simulink model "obliczeniaOffline"  (R2013a)
settings: Solver=FixedStepDiscrete  StartTime=0  StopTime=15  FixedStep=0.0025  RelTol=1e-3
InitFcn:
  | InitFcn
values from neighbouring files (symbols this model uses):
  accBias = zeros(3,1)    [InitFcn.m]
  accGain = accGain.*(9.81/9.761)    [InitFcn.m]
  gyroBias = zeros(3,1)    [InitFcn.m]
  gyroGain = ones(3,1)    [InitFcn.m]
  index = 1    [InitFcn.m]
  magBias = [(743-502);(743-507);(579-516)]/2    [InitFcn.m]
  magGainM = W_inverted    [InitFcn.m]
  usrednien = 5    [InitFcn.m]
undefined symbols (not defined in the file or in its folder): dfilt, DiscIntNeverNeededParam, eul_0, fdesignblkfcn, gcbh
libraries: dspstat3 x12, aerolibconvert2 x9, aerolibobsolete x7, aerolibtransform2 x4, dspmtrx3 x3, aerolibutil x3, dspsigops x1, dspsrcs4 x1, dsparch4 x1
settings Model: Creator=Antonio  LastModifiedBy=Antonio
settings SolverCC: AutoInsertRateTranBlk=on  InsertRTBMode=Always
settings OptimizationCC: LocalBlockOutputs=off  SimCompilerOptimization=On
settings SFSimCC: SFSimEnableDebug=off
settings RTWCC: RTWCompilerOptimization=On

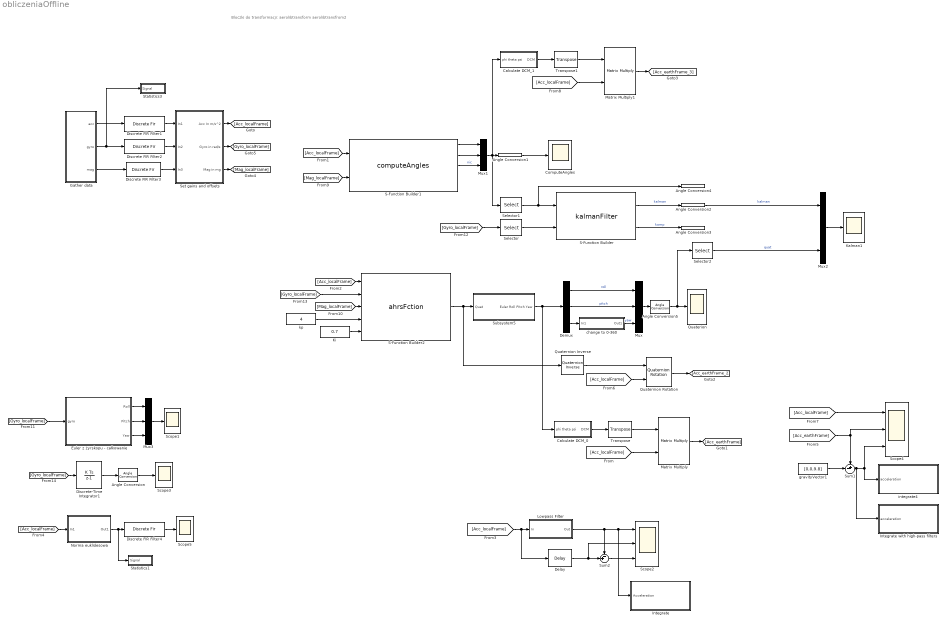
== system obliczeniaOffline ==
  note: Bloczki do transformacji:
      | aerolibtransform
      | aerolibtransfrom2
  " Set gains and offsets" : Subsystem
  Angle Conversion{,1..5} (6 alike) : aerolibconvert2/Angle Conversion  IU=rad  OU=deg
  Calculate DCM_0 : Subsystem
  Calculate DCM_1 : Subsystem
  ComputeAngles : Scope
      settings: TickLabels=on  ShowLegends=on  TimeRange=30  YMin=-125  YMax=375  SaveName=ScopeData3
  Delay : dspsigops/Delay  dly_unit=Samples  delay=0  ic_detail=off  dif_ic_for_ch=off  dif_ic_for_dly=off  ic=0  reset_popup=None
  Demux : Demux  Outputs=3
  Discrete FIR Filter1 : DiscreteFir  Coefficients=ones(1,usrednien)/usrednien
  Discrete FIR Filter2 : DiscreteFir  Coefficients=ones(1,usrednien)/usrednien
  Discrete FIR Filter3 : DiscreteFir  Coefficients=ones(1,usrednien)/usrednien
  Discrete FIR Filter4 : DiscreteFir  Coefficients=ones(1,15)/15
  Discrete-Time Integrator1 : DiscreteIntegrator  SampleTime=-1  ICPrevOutput=DiscIntNeverNeededParam  ICPrevScaledInput=DiscIntNeverNeededParam
  Euler z żyrskopu - całkowanie : Subsystem
  Gather data : Subsystem
  Integrate : Subsystem
  Integrate with high-pass filters : Subsystem
  Kalman1 : Scope
      settings: ShowLegends=on  TimeRange=15  YMin=-10  YMax=180  SaveName=ScopeData5
  Ki : Constant  Value=0.7  OutDataTypeStr=single
  Lowpass Filter : Subsystem  DialogController=fdesignblkfcn  InitFcn=fdesignblkfcn(gcbh, {'InitFcn'});  mask(Lowpass Filter){}
      mask help: Design a lowpass filter
      settings: CopyFcn=fdesignblkfcn(gcbh, {'CopyFcn'});
      mask Help: helpview(mapfilelocation('dsp'), 'dsplowpassfilter');
      mask Display: disp('Lowpass')
  Matrix Multiply : Product  Multiplication=Matrix(*)
  Matrix Multiply1 : Product  Multiplication=Matrix(*)
  Mux{,1..3} (4 alike) : Mux  Inputs=3
  Norma euklidesowa : Subsystem
  Quaterion : Scope
      settings: ShowLegends=on  TimeRange=15  YMin=-25  YMax=375  SaveName=ScopeData4
  Quaternion Inverse : aerolibutil/Quaternion Inverse
  Quaternion Rotation : aerolibutil/Quaternion Rotation
  S-Function Builder : S-Function  InitFcn=try, set_param(gcb,'FunctionName','kalmanFilter'), end  FunctionName=kalmanFilter  Parameters=single(0.0025)  SFunctionModules=kalmanFilter_wrapper Kalman  EnableBusSupport=off  mask(S-Function Builder){}
      mask help: Simulink:masks:SFunctionBuilder_MD
      mask init:
      | val = [[.9  0.75 0.75 1 1 .9 .9 1]',[1 1 0.75 0.75 .9 .9 1 .9]'];try , sys = get_param(gcb,'SfunBuilderFcnName');if isempty(sys), sys = get_param(gcb,'FunctionName'); end,catch, sys = get_param(gcb,'FunctionName'); end
      settings: CopyFcn=set_param(gcbh,'LinkStatus','none')  PreSaveFcn=try, set_param(gcb,'FunctionName','kalmanFilter'), end  OpenFcn=sfunctionwizard(gcbh)
      mask Display: plot(val(:,1),val(:,2)),disp(sys), port_label('input',1,'newAngleIn'), port_label('input',2,'newRateIn'), port_label('output',1,'angleOut'), port_label('output',2,'compAngleOut')
  S-Function Builder1 : S-Function  InitFcn=try, set_param(gcb,'FunctionName','computeAngles'), end  FunctionName=computeAngles  SFunctionModules=computeAngles_wrapper angles  EnableBusSupport=off  mask(S-Function Builder){}
      mask help: Simulink:masks:SFunctionBuilder_MD
      mask init: same as obliczeniaOffline/S-Function Builder
      settings: CopyFcn=set_param(gcbh,'LinkStatus','none')  PreSaveFcn=try, set_param(gcb,'FunctionName','computeAngles'), end  OpenFcn=sfunctionwizard(gcbh)
      mask Display: plot(val(:,1),val(:,2)),disp(sys), port_label('input',1,'accelerometerIn'), port_label('input',2,'magnetometerIn'), port_label('output',1,'XRollAngleOut'), port_label('output',2,'YPitchAngleOut'), port_label('output',3,'ZYawAngleOut'), port_label('output',4,'ZYawAngleFlatOut'), port_label('output',5,'TiltAngleOut')
  S-Function Builder2 : S-Function  InitFcn=try, set_param(gcb,'FunctionName','ahrsFction'), end  FunctionName=ahrsFction  SFunctionModules=ahrsFction_wrapper artykul MahonyAHRS  EnableBusSupport=off  mask(S-Function Builder){}
      mask help: Simulink:masks:SFunctionBuilder_MD
      mask init: same as obliczeniaOffline/S-Function Builder
      settings: CopyFcn=set_param(gcbh,'LinkStatus','none')  PreSaveFcn=try, set_param(gcb,'FunctionName','ahrsFction'), end  OpenFcn=sfunctionwizard(gcbh)
      mask Display: plot(val(:,1),val(:,2)),disp(sys), port_label('input',1,'accIn'), port_label('input',2,'gyroIn'), port_label('input',3,'magIn'), port_label('input',4,'Kp'), port_label('input',5,'Ki'), port_label('output',1,'quat')
  Scope1 : Scope
      settings: ShowLegends=on  TimeRange=60  YMin=-3  YMax=3
  Scope2 : Scope  NumInputPorts=3
      settings: ShowLegends=on  TimeRange=15  YMin=-2~-5~-4  YMax=10~15~10  SaveName=ScopeData2
  Scope3 : Scope
      settings: ShowLegends=on  TimeRange=60  YMin=-350  YMax=50  SaveName=ScopeData6
  Scope4 : Scope  NumInputPorts=3
      settings: ShowLegends=on  TimeRange=15  YMin=-2.03431~-2~-2  YMax=11.8546~11~1.75  SaveName=ScopeData8
  Scope5 : Scope
      settings: ShowLegends=on  TimeRange=60  YMin=2  YMax=11  SaveName=ScopeData11
  Selector : Selector  InputPortWidth=3  IndexOptions=Index vector (dialog)  Indices=[index]  OutputSizes=1
  Selector1 : Selector  InputPortWidth=3  IndexOptions=Index vector (dialog)  Indices=[index]  OutputSizes=1
  Selector2 : Selector  InputPortWidth=3  IndexOptions=Index vector (dialog)  Indices=[index]  OutputSizes=1
  Statistics1 : Subsystem
  Statistics3 : Subsystem
  Subsystem5 : Subsystem
  Sum1 : Sum  Inputs=+-|
  Sum2 : Sum  Inputs=-+|
  Transpose : dspmtrx3/Transpose  Hermitian=off  overflowFlag=off
  Transpose1 : dspmtrx3/Transpose  Hermitian=off  overflowFlag=off
  change to 0-360 : Subsystem
  gravityVector1 : Constant  Value=[0,0,9.8]
  integrate4 : Subsystem
  kp : Constant  Value=4  OutDataTypeStr=single
  wires:
  Selector/1 -> S-Function Builder/2
  Gather data/1(acc) -> Discrete FIR Filter1/1
  Gather data/2(gyro) -> Discrete FIR Filter2/1, Statistics3/1(Signal)
  Gather data/3(mag) -> Discrete FIR Filter3/1
  Discrete FIR Filter2/1 -> " Set gains and offsets"/2(In2)
  Discrete FIR Filter3/1 -> " Set gains and offsets"/3(In3)
  Mux2/1 -> Kalman1/1
  Mux/1 -> Angle Conversion5/1
  Demux/3 -> change to 0-360/1(In1)
  change to 0-360/1(Out1) -> Mux/3  "yaw"
  Demux/2 -> Mux/2  "pitch"
  Demux/1 -> Mux/1  "roll"
  S-Function Builder1/2 -> Mux1/2
  S-Function Builder1/3 -> Mux1/3  "nic"
  S-Function Builder1/1 -> Mux1/1
  Selector1/1 -> Angle Conversion4/1, S-Function Builder/1
  Angle Conversion1/1 -> ComputeAngles/1
  Euler z żyrskopu - całkowanie/1(Roll) -> Mux3/1
  Euler z żyrskopu - całkowanie/2(Pitch) -> Mux3/2
  Euler z żyrskopu - całkowanie/3(Yaw) -> Mux3/3
  Mux3/1 -> Scope1/1
  Selector2/1 -> Mux2/3  "quat"
  S-Function Builder/2 -> Angle Conversion3/1  "komp"
  S-Function Builder/1 -> Angle Conversion2/1  "kalman"
  Discrete-Time Integrator1/1 -> Angle Conversion/1
  Angle Conversion/1 -> Scope3/1
  Mux1/1 -> Calculate DCM_1/1(phi theta psi), Selector1/1, Angle Conversion1/1
  kp/1 -> S-Function Builder2/4
  Ki/1 -> S-Function Builder2/5
  Calculate DCM_0/1(DCM) -> Transpose/1
  Subsystem5/1(Euler Roll Pitch Yaw) -> Demux/1, Calculate DCM_0/1(phi theta psi)
  Angle Conversion2/1 -> Mux2/1  "kalman"
  Transpose/1 -> Matrix Multiply/1
  [Acc_localFrame] -> Matrix Multiply/2
  gravityVector1/1 -> Sum1/2
  Matrix Multiply/1 -> [Acc_earthFrame]
  S-Function Builder2/1 -> Quaternion Inverse/1, Subsystem5/1(Quat)
  [Acc_localFrame] -> S-Function Builder1/1
  [Acc_localFrame] -> S-Function Builder2/1
  Quaternion Inverse/1 -> Quaternion Rotation/1
  Sum2/1 -> Scope2/3
  [Acc_localFrame] -> Lowpass Filter/1(In), Delay/1
  Delay/1 -> Scope2/2, Sum2/2
  Norma euklidesowa/1(Out1) -> Statistics1/1(Signal), Discrete FIR Filter4/1
  [Acc_localFrame] -> Norma euklidesowa/1(In1)
  Angle Conversion5/1 -> Selector2/1, Quaterion/1
  [Acc_earthFrame] -> Sum1/1, Scope4/2
  [Acc_localFrame] -> Quaternion Rotation/2
  Quaternion Rotation/1 -> [Acc_earthFrame_2]
  [Acc_localFrame] -> Scope4/1
  Discrete FIR Filter1/1 -> " Set gains and offsets"/1(In1)
  Lowpass Filter/1(Out) -> Integrate/1(Acceleration), Scope2/1, Sum2/1
  Discrete FIR Filter4/1 -> Scope5/1
  " Set gains and offsets"/1(Acc In m/s^2) -> [Acc_localFrame]
  Sum1/1 -> Integrate with high-pass filters/1(acceleration), integrate4/1(acceleration), Scope4/3
  Calculate DCM_1/1(DCM) -> Transpose1/1
  Transpose1/1 -> Matrix Multiply1/1
  [Acc_localFrame] -> Matrix Multiply1/2
  Matrix Multiply1/1 -> [Acc_earthFrame_3]
  " Set gains and offsets"/3(Mag in mg) -> [Mag_localFrame]
  [Mag_localFrame] -> S-Function Builder1/2
  [Mag_localFrame] -> S-Function Builder2/3
  " Set gains and offsets"/2(Gyro in rad/s) -> [Gyro_localFrame]
  [Gyro_localFrame] -> Euler z żyrskopu - całkowanie/1(gyro)
  [Gyro_localFrame] -> Selector/1
  [Gyro_localFrame] -> S-Function Builder2/2
  [Gyro_localFrame] -> Discrete-Time Integrator1/1

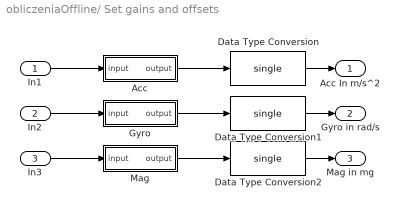
== system obliczeniaOffline/ Set gains and offsets ==
  In1 : Inport
  In2 : Inport  Port=2
  In3 : Inport  Port=3
  Acc : Subsystem
  Data Type Conversion : DataTypeConversion  OutDataTypeStr=single
  Data Type Conversion1 : DataTypeConversion  OutDataTypeStr=single
  Data Type Conversion2 : DataTypeConversion  OutDataTypeStr=single
  Gyro : Subsystem
  Mag : Subsystem
  Acc In m/s^2 : Outport
  Gyro in rad/s : Outport  Port=2
  Mag in mg : Outport  Port=3
  wires:
  Gyro/1(output) -> Data Type Conversion1/1
  In3/1 -> Mag/1(input)
  In2/1 -> Gyro/1(input)
  Acc/1(output) -> Data Type Conversion/1
  In1/1 -> Acc/1(input)
  Mag/1(output) -> Data Type Conversion2/1
  Data Type Conversion/1 -> Acc In m/s^2/1
  Data Type Conversion1/1 -> Gyro in rad/s/1
  Data Type Conversion2/1 -> Mag in mg/1

== system obliczeniaOffline/Calculate DCM_0 ==
  phi theta psi : Inport
  Rotation Angles to Direction Cosine Matrix : aerolibtransform2/Rotation Angles to Direction Cosine Matrix  rotationOrder=ZYX
  Selector : Selector  InputPortWidth=3  IndexOptions=Index vector (dialog)  Indices=[3 2 1]  OutputSizes=1
  DCM : Outport
  wires:
  Selector/1 -> Rotation Angles to Direction Cosine Matrix/1
  phi theta psi/1 -> Selector/1
  Rotation Angles to Direction Cosine Matrix/1 -> DCM/1

== system obliczeniaOffline/Calculate DCM_1 ==
  phi theta psi : Inport
  Rotation Angles to Direction Cosine Matrix : aerolibtransform2/Rotation Angles to Direction Cosine Matrix  rotationOrder=ZYX
  Selector : Selector  InputPortWidth=3  IndexOptions=Index vector (dialog)  Indices=[3 2 1]  OutputSizes=1
  DCM : Outport
  wires:
  Selector/1 -> Rotation Angles to Direction Cosine Matrix/1
  phi theta psi/1 -> Selector/1
  Rotation Angles to Direction Cosine Matrix/1 -> DCM/1

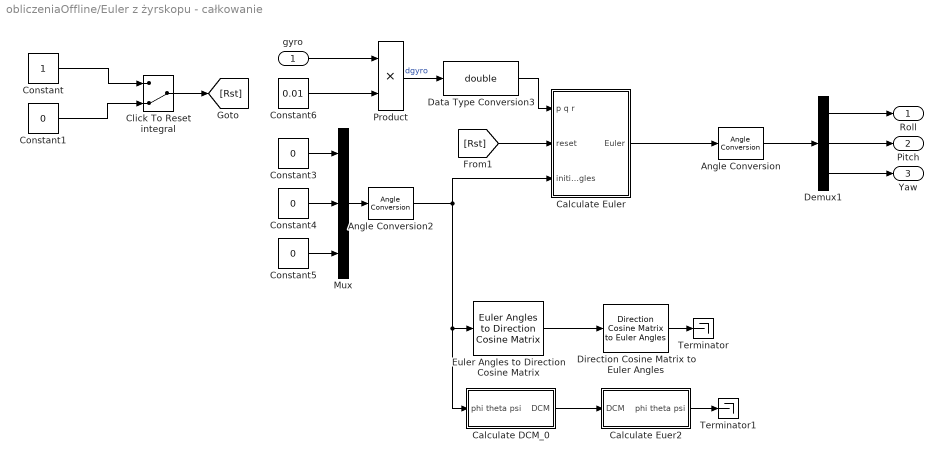
== system obliczeniaOffline/Euler z żyrskopu - całkowanie ==
  gyro : Inport
  Angle Conversion : aerolibconvert2/Angle Conversion  IU=rad  OU=deg
  Angle Conversion2 : aerolibconvert2/Angle Conversion  IU=deg  OU=rad
  Calculate DCM_0 : Subsystem
  Calculate Euer2 : Subsystem
  Calculate Euler : Subsystem
  Click To Reset integral : ManualSwitch  CurrentSetting=0
  Constant : Constant
  Constant{1,3..5} (4 alike) : Constant  Value=0
  Constant6 : Constant  Value=0.01  OutDataTypeStr=single
  Data Type Conversion3 : DataTypeConversion  OutDataTypeStr=double
  Demux1 : Demux  Outputs=3
  Direction Cosine Matrix to Euler Angles : aerolibobsolete/Direction Cosine Matrix to Euler Angles
  Euler Angles to Direction Cosine Matrix : aerolibobsolete/Euler Angles to  Direction Cosine Matrix
  Mux : Mux  Inputs=3
  Product : Product
  Terminator : Terminator
  Terminator1 : Terminator
  Roll : Outport
  Pitch : Outport  Port=2
  Yaw : Outport  Port=3
  wires:
  Constant/1 -> Click To Reset integral/1
  Constant1/1 -> Click To Reset integral/2
  Click To Reset integral/1 -> [Rst]
  Calculate Euler/1(Euler) -> Angle Conversion/1
  Demux1/2 -> Pitch/1
  Demux1/1 -> Roll/1
  Demux1/3 -> Yaw/1
  Angle Conversion/1 -> Demux1/1
  Constant3/1 -> Mux/1
  Constant4/1 -> Mux/2
  Constant5/1 -> Mux/3
  Mux/1 -> Angle Conversion2/1
  [Rst] -> Calculate Euler/2(reset)
  Angle Conversion2/1 -> Calculate Euler/3(initialAngles), Calculate DCM_0/1(phi theta psi), Euler Angles to Direction Cosine Matrix/1
  Constant6/1 -> Product/2
  Product/1 -> Data Type Conversion3/1  "dgyro"
  Euler Angles to Direction Cosine Matrix/1 -> Direction Cosine Matrix to Euler Angles/1
  Calculate DCM_0/1(DCM) -> Calculate Euer2/1(DCM)
  Data Type Conversion3/1 -> Calculate Euler/1(p q r)
  gyro/1 -> Product/1
  Direction Cosine Matrix to Euler Angles/1 -> Terminator/1
  Calculate Euer2/1(phi theta psi) -> Terminator1/1

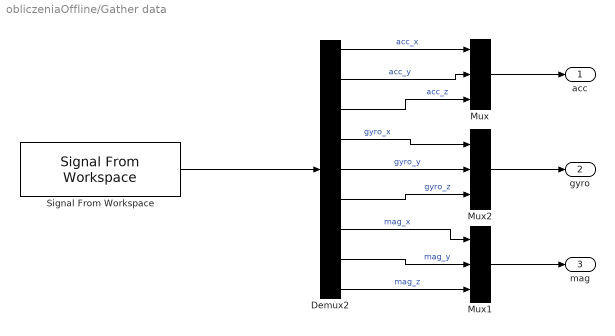
== system obliczeniaOffline/Gather data ==
  Demux2 : Demux  Outputs=9
  Mux : Mux  Inputs=3
  Mux1 : Mux  Inputs=3
  Mux2 : Mux  Inputs=3
  Signal From Workspace : dspsrcs4/Signal From Workspace  X=measurement  Ts=0.0025  nsamps=1  OutputAfterFinalValue=Holding final value  ignoreOrWarnInputAndFrameLengths=off
  acc : Outport
  gyro : Outport  Port=2
  mag : Outport  Port=3
  wires:
  Demux2/1 -> Mux/1  "acc_x"
  Demux2/2 -> Mux/2  "acc_y"
  Demux2/3 -> Mux/3  "acc_z"
  Mux/1 -> acc/1
  Demux2/5 -> Mux2/2  "gyro_y"
  Demux2/4 -> Mux2/1  "gyro_x"
  Demux2/6 -> Mux2/3  "gyro_z"
  Mux2/1 -> gyro/1
  Demux2/7 -> Mux1/1  "mag_x"
  Demux2/8 -> Mux1/2  "mag_y"
  Demux2/9 -> Mux1/3  "mag_z"
  Mux1/1 -> mag/1
  Signal From Workspace/1 -> Demux2/1

== system obliczeniaOffline/Integrate ==
  Acceleration : Inport
  Discrete-Time Integrator2 : DiscreteIntegrator  gainval=1  SampleTime=-1  ICPrevOutput=DiscIntNeverNeededParam  ICPrevScaledInput=DiscIntNeverNeededParam
  Discrete-Time Integrator3 : DiscreteIntegrator  gainval=1  SampleTime=-1  ICPrevOutput=DiscIntNeverNeededParam  ICPrevScaledInput=DiscIntNeverNeededParam
  Product : Product
  Step : Step  Time=5
  m to cm : Gain  Gain=100
  pozycja : Scope  NumInputPorts=3
      settings: ShowLegends=on  TimeRange=15  YMin=-15~-500~-0.4  YMax=15~4750~0.05  SaveName=ScopeData10
  wires:
  Discrete-Time Integrator2/1 -> pozycja/2, Discrete-Time Integrator3/1  "velocity"
  Discrete-Time Integrator3/1 -> pozycja/3  "position"
  Product/1 -> m to cm/1
  Acceleration/1 -> Product/1
  Step/1 -> Product/2
  m to cm/1 -> Discrete-Time Integrator2/1, pozycja/1

== system obliczeniaOffline/Integrate with high-pass filters ==
  acceleration : Inport
  Discrete-Time Integrator2 : DiscreteIntegrator  gainval=1  SampleTime=-1  ICPrevOutput=DiscIntNeverNeededParam  ICPrevScaledInput=DiscIntNeverNeededParam
  Discrete-Time Integrator3 : DiscreteIntegrator  gainval=0.5  SampleTime=-1  ICPrevOutput=DiscIntNeverNeededParam  ICPrevScaledInput=DiscIntNeverNeededParam
  Highpass Filter2 : Subsystem  DialogController=fdesignblkfcn  InitFcn=fdesignblkfcn(gcbh, {'InitFcn'});  mask(Highpass Filter){}
      mask help: Design a highpass filter
      settings: CopyFcn=fdesignblkfcn(gcbh, {'CopyFcn'});
      mask Help: helpview(mapfilelocation('dsp'), 'dsphighpassfilter');
      mask Display: disp('Highpass')
  Product : Product
  Step : Step  Time=5
  m to cm : Gain  Gain=100
  pozycja : Scope  NumInputPorts=3
      settings: ShowLegends=on  TimeRange=15  YMin=-150~-25~-30  YMax=150~25~20  SaveName=ScopeData10
  wires:
  Discrete-Time Integrator2/1 -> pozycja/2, Discrete-Time Integrator3/1  "velocity"
  Discrete-Time Integrator3/1 -> pozycja/3  "position"
  Product/1 -> m to cm/1
  acceleration/1 -> Product/1
  Step/1 -> Product/2
  Highpass Filter2/1(Out) -> pozycja/1, Discrete-Time Integrator2/1
  m to cm/1 -> Highpass Filter2/1(In)

== system obliczeniaOffline/Lowpass Filter ==
  In : Inport
  Generated Filter Block : DiscreteFir  Tag=BlockMethodSubSystem  Coefficients=[0.00050680699585200345 1.8104768139348693e-05 1.6977561331381059e-05 1.4833633469184346e-05 1.1634485977210355e-05 7.3434816185162684e-06 1.925238505602481e-06 -4.6554062756843208e-06 -1.2428942588863933e-05 -2.14243220317547e-05 -3.1665536877958055e-05 -4.3173212468487982e-05 -5.596345481140389e-05 -7.0045256722031624e-05 -8.5422243813193955e-05 -0.0001020913503340876 -0.00012004374546061746 -0.0001392619546353783 -0.00015972622688413584 -0.00018138836919694775 -0.00020423491202698217 -0.00022818978603687275 -0.00025320269989232124 -0.00027921558906226688 -0.00030614886036985707 -0.00033391218088171478 -0.00036241524341515939 -0.00039155711714154967 -0.00042123049572248105 -0.00045131620561162018 -0.00048168727910416389 -0.00051221020993199337 -0.00054274521301832886 -0.00057314784243304084 -0.00060326880695485527 -0.00063295356901068699 -0.00066204167658164611 -0.00069037270007361678 -0.00071777933332873526 -0.00074410555802311438 -0.00076918180057893579 -0.00079284492083031837 -0.00081493914228260192 -0.00083530657953818509 -0.00085378919210934404 -0.00087024715251888445 -0.00088453633553146611 -0.00089652433072802298 -0.00090608418959002091 -0.00091310030908900691 -0.00091746820875369787 -0.00091909427196526061 -0.00091789573503021709 -0.00091380214009601022 -0.00090675563447802381 -0.00089671236011365518 -0.00088364731133413999 -0.00086754948936208873 -0.00084842749881238876 -0.00082629818291407955 -0.00080119748719947067 -0.00077319086865142021 -0.0007423606677744815 -0.00070877954903689048 -0.00067258226676091047 -0.00063388601583306409 -0.00059284204523740128 -0.00054961325206677003 -0.00050437902638090885 -0.00045733140230810318 -0.00040867457706862047 -0.00035862264400760783 -0.00030740039285116294 -0.00025524021333557913 -0.00020238061194014591 -0.00014906827871743485 -9.555603919256272e-05 -4.2109642615560943e-05 1.0990394190089968e-05 6.3432131552027015e-05 0.00011481508771645329 0.000163929526711354 0.00021337941369384917 0.00026014518432284408 0.00030496071711733048 0.00034749727121142219 0.00038749962497370752 0.00042472979420425259 0.00045896558094866979 0.00048999762759601795 0.00051763444976912288 0.00054170106937079287 0.00056204277991718878 0.00057852591164379548 0.00059103671920925928 0.00059948483928015488 0.00060380313045349618 0.00060395022421946181 0.0005999086230995391 0.00059169306814376116 0.00057931861944241988 0.00056288200358844227 0.00054243478381470699 0.00051810065614346363 0.00049002865769549658 0.00045837773939839727 0.0004233288051232909 0.00038509540043196559 0.00034391229856337252 0.00030003785456418733 0.00025374627222805494 0.0002053296340389396 0.00015509716876202419 0.00010337338110347834 5.0497602022540693e-05 -3.1789803530603983e-06 -5.7296714938403917e-05 -0.00011149165215694587 -0.00016539253821891225 -0.00021863218629743133 -0.00027082953146300635 -0.0003216221132869809 -0.00037064610713815347 -0.00041754058093965694 -0.00046196133091381565 -0.00050358116726620307 -0.00054207560146992545 -0.00057714811813586371 -0.00060851810603824888 -0.00063593013978642055 -0.00065915071230361502 -0.00067797096142335322 -0.00069220947241619779 -0.00070171458496094436 -0.00070636537888095789 -0.00070607362183796652 -0.00070078440447933759 -0.00069047251380168991 -0.00067514898155686962 -0.00065485547577851465 -0.0006296782561620325 -0.00059973710746372762 -0.00056517563643030462 -0.00052617404653279305 -0.00048297031526965364 -0.00043579580170031166 -0.00038494458296995683 -0.00033072396635073088 -0.00027347214432053829 -0.00021354989195547714 -0.00015134089229504571 -8.7248797179902441e-05 -2.1695978491134758e-05 4.4880429387894182e-05 0.00011202804206761498 0.00017927981156929496 0.00024615815775456187 0.00031217479280710493 0.00037684128493064596 0.00043967486237110029 0.00050021947128286873 0.0005580848283111197 0.00061307792246632106 0.0006639966539519446 0.00071116167118856575 0.000753898713209556 0.00079188230416504021 0.00082478164102509045 0.0008522956280890945 0.00087415501109185589 ...(+15061 chars)]
  Out : Outport
  wires:
  In/1 -> Generated Filter Block/1
  Generated Filter Block/1 -> Out/1

== system obliczeniaOffline/Norma euklidesowa ==
  In1 : Inport
  Matrix Multiply1 : Product  Multiplication=Matrix(*)
  Sqrt : Sqrt  SaturateOnIntegerOverflow=on
  Transpose1 : dspmtrx3/Transpose  Hermitian=off  overflowFlag=off
  Out1 : Outport
  wires:
  Transpose1/1 -> Matrix Multiply1/1
  In1/1 -> Matrix Multiply1/2, Transpose1/1
  Matrix Multiply1/1 -> Sqrt/1
  Sqrt/1 -> Out1/1

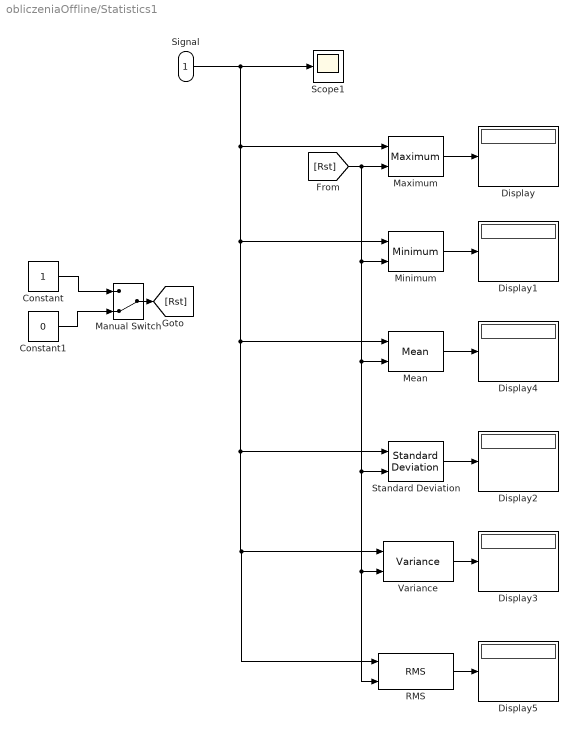
== system obliczeniaOffline/Statistics1 ==
  Signal : Inport
  Constant : Constant
  Constant1 : Constant  Value=0
  Display{,1..5} (6 alike) : Display
  Manual Switch : ManualSwitch  CurrentSetting=0
  Maximum : dspstat3/Maximum  fcn=Running  reset=Either edge  indexBase=One  operateOver=Each column  Dimension=1  colComp=on  operation=maximum  roiEnable=off  roiType=Rectangles  roiPortion=Entire ROI  roiOutput=Individual statistics for each ROI  roiFlag=off  accumDataTypeStr=Inherit: Same as product output  accumLastDataTypeStr=Inherit: Same as product output  roundingMode=Floor  overflowMode=off
  Mean : dspstat3/Mean  run=on  reset_popup=Either edge  directionMode=Each column  dimension=1  treatSBRowAsCol=on  roiEnable=off  roiType=Rectangles  roiPortion=Entire ROI  roiOutput=Individual statistics for each ROI  roiFlag=off  outputDataTypeStr=Inherit: Same as accumulator  outputLastDataTypeStr=Inherit: Same as accumulator  outputMin=[]  outputMax=[]  roundingMode=Floor  overflowMode=off
  Minimum : dspstat3/Minimum  fcn=Running  reset=Either edge  indexBase=One  operateOver=Each column  Dimension=1  colComp=on  operation=minimum  roiEnable=off  roiType=Rectangles  roiPortion=Entire ROI  roiOutput=Individual statistics for each ROI  roiFlag=off  roundingMode=Floor  overflowMode=off
  RMS : dspstat3/RMS  run=on  reset_popup=Either edge  directionMode=Each column  dimension=1  treatSBRowAsCol=on
  Scope1 : Scope
      settings: ShowLegends=on  TimeRange=50  YMin=-40000  YMax=40000
  Standard Deviation : dspstat3/Standard Deviation  run=on  reset_popup=Either edge  directionMode=Each column  dimension=1  treatSBRowAsCol=on  roiEnable=off  roiType=Rectangles  roiPortion=Entire ROI  roiOutput=Individual statistics for each ROI  roiFlag=off
  Variance : dspstat3/Variance  run=on  reset_popup=Either edge  directionMode=Each column  dimension=1  treatSBRowAsCol=on  roiEnable=off  roiType=Rectangles  roiPortion=Entire ROI  roiOutput=Individual statistics for each ROI  roiFlag=off  roundingMode=Floor  overflowMode=off
  wires:
  Variance/1 -> Display3/1
  Constant/1 -> Manual Switch/1
  Standard Deviation/1 -> Display2/1
  Constant1/1 -> Manual Switch/2
  Minimum/1 -> Display1/1
  Manual Switch/1 -> [Rst]
  Maximum/1 -> Display/1
  Signal/1 -> Scope1/1, Mean/1, RMS/1, Variance/1, Standard Deviation/1, Minimum/1, Maximum/1
  Mean/1 -> Display4/1
  [Rst] -> Minimum/2, Mean/2, RMS/2, Variance/2, Standard Deviation/2, Maximum/2
  RMS/1 -> Display5/1

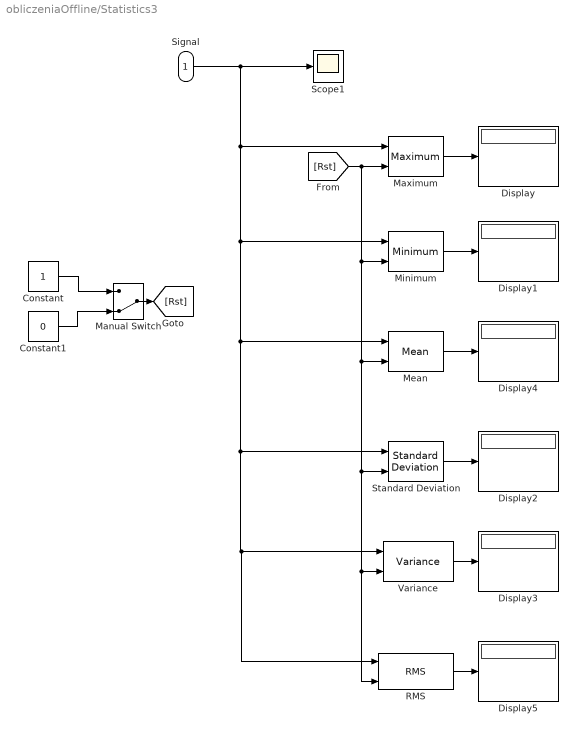
== system obliczeniaOffline/Statistics3 ==
  Signal : Inport
  Constant : Constant
  Constant1 : Constant  Value=0
  Display{,1..5} (6 alike) : Display
  Manual Switch : ManualSwitch  CurrentSetting=0
  Maximum : dspstat3/Maximum  fcn=Running  reset=Either edge  indexBase=One  operateOver=Each column  Dimension=1  colComp=on  operation=maximum  roiEnable=off  roiType=Rectangles  roiPortion=Entire ROI  roiOutput=Individual statistics for each ROI  roiFlag=off  accumDataTypeStr=Inherit: Same as product output  accumLastDataTypeStr=Inherit: Same as product output  roundingMode=Floor  overflowMode=off
  Mean : dspstat3/Mean  run=on  reset_popup=Either edge  directionMode=Each column  dimension=1  treatSBRowAsCol=on  roiEnable=off  roiType=Rectangles  roiPortion=Entire ROI  roiOutput=Individual statistics for each ROI  roiFlag=off  outputDataTypeStr=Inherit: Same as accumulator  outputLastDataTypeStr=Inherit: Same as accumulator  outputMin=[]  outputMax=[]  roundingMode=Floor  overflowMode=off
  Minimum : dspstat3/Minimum  fcn=Running  reset=Either edge  indexBase=One  operateOver=Each column  Dimension=1  colComp=on  operation=minimum  roiEnable=off  roiType=Rectangles  roiPortion=Entire ROI  roiOutput=Individual statistics for each ROI  roiFlag=off  roundingMode=Floor  overflowMode=off
  RMS : dspstat3/RMS  run=on  reset_popup=Either edge  directionMode=Each column  dimension=1  treatSBRowAsCol=on
  Scope1 : Scope
      settings: ShowLegends=on  TimeRange=50  YMin=-40000  YMax=40000
  Standard Deviation : dspstat3/Standard Deviation  run=on  reset_popup=Either edge  directionMode=Each column  dimension=1  treatSBRowAsCol=on  roiEnable=off  roiType=Rectangles  roiPortion=Entire ROI  roiOutput=Individual statistics for each ROI  roiFlag=off
  Variance : dspstat3/Variance  run=on  reset_popup=Either edge  directionMode=Each column  dimension=1  treatSBRowAsCol=on  roiEnable=off  roiType=Rectangles  roiPortion=Entire ROI  roiOutput=Individual statistics for each ROI  roiFlag=off  roundingMode=Floor  overflowMode=off
  wires:
  Variance/1 -> Display3/1
  Constant/1 -> Manual Switch/1
  Standard Deviation/1 -> Display2/1
  Constant1/1 -> Manual Switch/2
  Minimum/1 -> Display1/1
  Manual Switch/1 -> [Rst]
  Maximum/1 -> Display/1
  Signal/1 -> Scope1/1, Mean/1, RMS/1, Variance/1, Standard Deviation/1, Minimum/1, Maximum/1
  Mean/1 -> Display4/1
  [Rst] -> Minimum/2, Mean/2, RMS/2, Variance/2, Standard Deviation/2, Maximum/2
  RMS/1 -> Display5/1

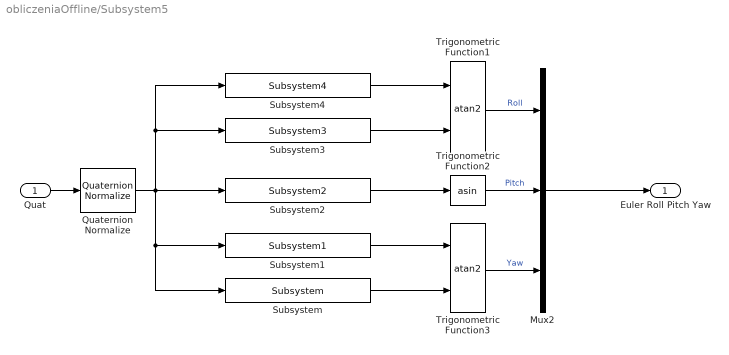
== system obliczeniaOffline/Subsystem5 ==
  Quat : Inport
  Mux2 : Mux  Inputs=3
  Quaternion Normalize : aerolibutil/Quaternion Normalize
  Subsystem : aerolibobsolete/Quaternions to Euler Angles/Subsystem
  Subsystem1 : aerolibobsolete/Quaternions to Euler Angles/Subsystem1
  Subsystem2 : aerolibobsolete/Quaternions to Euler Angles/Subsystem2
  Subsystem3 : aerolibobsolete/Quaternions to Euler Angles/Subsystem3
  Subsystem4 : aerolibobsolete/Quaternions to Euler Angles/Subsystem4
  Trigonometric Function1 : Trigonometry  Operator=atan2
  Trigonometric Function2 : Trigonometry  Operator=asin
  Trigonometric Function3 : Trigonometry  Operator=atan2
  Euler Roll Pitch Yaw : Outport  InitialOutput=0
  wires:
  Trigonometric Function1/1 -> Mux2/1  "Roll"
  Subsystem/1 -> Trigonometric Function3/2
  Subsystem1/1 -> Trigonometric Function3/1
  Trigonometric Function3/1 -> Mux2/3  "Yaw"
  Subsystem3/1 -> Trigonometric Function1/2
  Subsystem4/1 -> Trigonometric Function1/1
  Subsystem2/1 -> Trigonometric Function2/1
  Trigonometric Function2/1 -> Mux2/2  "Pitch"
  Quaternion Normalize/1 -> Subsystem2/1, Subsystem4/1, Subsystem3/1, Subsystem1/1, Subsystem/1
  Quat/1 -> Quaternion Normalize/1
  Mux2/1 -> Euler Roll Pitch Yaw/1

== system obliczeniaOffline/change to 0-360 ==
  In1 : Inport
  Bias : Bias  Bias=2*pi
  Switch : Switch  Criteria=u2 > Threshold  OutDataTypeStr=Inherit: Inherit via back propagation
  Out1 : Outport  OutDataTypeStr=single
  wires:
  In1/1 -> Bias/1, Switch/2, Switch/1
  Bias/1 -> Switch/3
  Switch/1 -> Out1/1

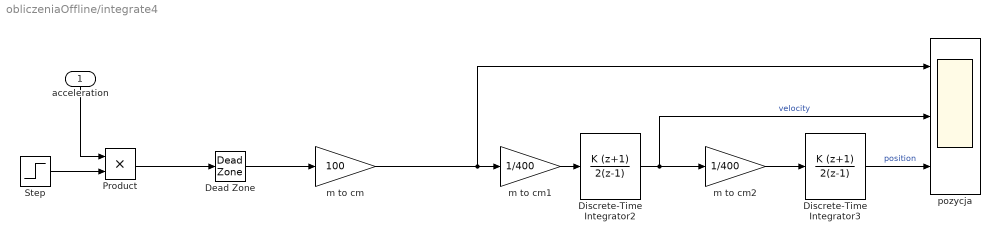
== system obliczeniaOffline/integrate4 ==
  acceleration : Inport
  Dead Zone : DeadZone  LowerValue=-0.2  UpperValue=0.2  SaturateOnIntegerOverflow=on
  Discrete-Time Integrator2 : DiscreteIntegrator  IntegratorMethod=Accumulation: Trapezoidal  gainval=1  SampleTime=-1  ICPrevOutput=DiscIntNeverNeededParam  ICPrevScaledInput=DiscIntNeverNeededParam
  Discrete-Time Integrator3 : DiscreteIntegrator  IntegratorMethod=Accumulation: Trapezoidal  gainval=1  SampleTime=-1  ICPrevOutput=DiscIntNeverNeededParam  ICPrevScaledInput=DiscIntNeverNeededParam
  Product : Product
  Step : Step  Time=1.5
  m to cm : Gain  Gain=100
  m to cm1 : Gain  Gain=1/400
  m to cm2 : Gain  Gain=1/400
  pozycja : Scope  NumInputPorts=3
      settings: ShowLegends=on  TimeRange=15  YMin=-200~-10~-100  YMax=200~27.5~100  SaveName=ScopeData10
  wires:
  Discrete-Time Integrator2/1 -> pozycja/2, m to cm2/1  "velocity"
  Discrete-Time Integrator3/1 -> pozycja/3  "position"
  Product/1 -> Dead Zone/1
  acceleration/1 -> Product/1
  Step/1 -> Product/2
  m to cm/1 -> m to cm1/1, pozycja/1
  m to cm1/1 -> Discrete-Time Integrator2/1
  m to cm2/1 -> Discrete-Time Integrator3/1
  Dead Zone/1 -> m to cm/1

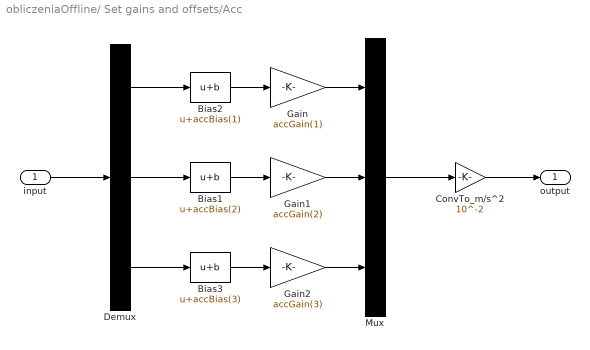
== system obliczeniaOffline/ Set gains and offsets/Acc ==
  input : Inport
  Bias1 : Bias  Bias=accBias(2)  SaturateOnIntegerOverflow=on
  Bias2 : Bias  Bias=accBias(1)  SaturateOnIntegerOverflow=on
  Bias3 : Bias  Bias=accBias(3)  SaturateOnIntegerOverflow=on
  ConvTo_m/s^2 : Gain  Gain=10^-2
  Demux : Demux  Outputs=3
  Gain : Gain  Gain=accGain(1)
  Gain1 : Gain  Gain=accGain(2)
  Gain2 : Gain  Gain=accGain(3)
  Mux : Mux  Inputs=3
  output : Outport
  wires:
  Mux/1 -> ConvTo_m/s^2/1
  input/1 -> Demux/1
  Gain1/1 -> Mux/2
  Gain2/1 -> Mux/3
  Demux/1 -> Bias2/1
  Bias2/1 -> Gain/1
  Gain/1 -> Mux/1
  Demux/2 -> Bias1/1
  Bias1/1 -> Gain1/1
  Demux/3 -> Bias3/1
  Bias3/1 -> Gain2/1
  ConvTo_m/s^2/1 -> output/1

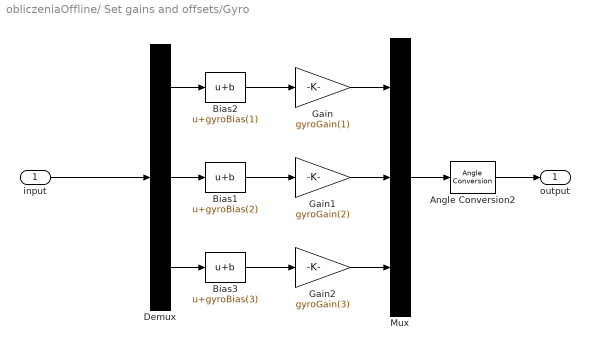
== system obliczeniaOffline/ Set gains and offsets/Gyro ==
  input : Inport
  Angle Conversion2 : aerolibconvert2/Angle Conversion  IU=deg  OU=rad
  Bias1 : Bias  Bias=gyroBias(2)  SaturateOnIntegerOverflow=on
  Bias2 : Bias  Bias=gyroBias(1)  SaturateOnIntegerOverflow=on
  Bias3 : Bias  Bias=gyroBias(3)  SaturateOnIntegerOverflow=on
  Demux : Demux  Outputs=3
  Gain : Gain  Gain=gyroGain(1)
  Gain1 : Gain  Gain=gyroGain(2)
  Gain2 : Gain  Gain=gyroGain(3)
  Mux : Mux  Inputs=3
  output : Outport
  wires:
  Bias1/1 -> Gain1/1
  Bias3/1 -> Gain2/1
  Demux/1 -> Bias2/1
  Bias2/1 -> Gain/1
  Demux/2 -> Bias1/1
  Demux/3 -> Bias3/1
  Gain1/1 -> Mux/2
  Gain2/1 -> Mux/3
  Gain/1 -> Mux/1
  Mux/1 -> Angle Conversion2/1
  input/1 -> Demux/1
  Angle Conversion2/1 -> output/1

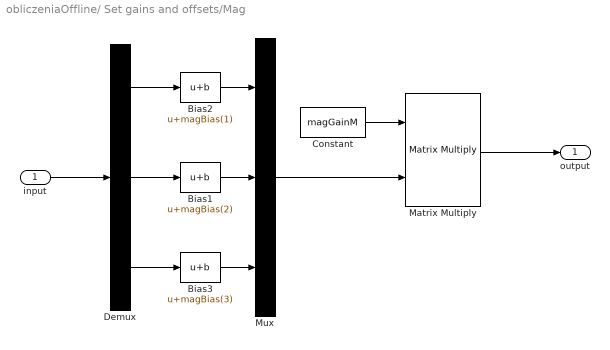
== system obliczeniaOffline/ Set gains and offsets/Mag ==
  input : Inport
  Bias1 : Bias  Bias=magBias(2)  SaturateOnIntegerOverflow=on
  Bias2 : Bias  Bias=magBias(1)  SaturateOnIntegerOverflow=on
  Bias3 : Bias  Bias=magBias(3)  SaturateOnIntegerOverflow=on
  Constant : Constant  Value=magGainM  OutDataTypeStr=single
  Demux : Demux  Outputs=3
  Matrix Multiply : Product  Multiplication=Matrix(*)
  Mux : Mux  Inputs=3
  output : Outport
  wires:
  input/1 -> Demux/1
  Bias1/1 -> Mux/2
  Bias3/1 -> Mux/3
  Demux/1 -> Bias2/1
  Bias2/1 -> Mux/1
  Demux/2 -> Bias1/1
  Demux/3 -> Bias3/1
  Mux/1 -> Matrix Multiply/2
  Constant/1 -> Matrix Multiply/1
  Matrix Multiply/1 -> output/1

== system obliczeniaOffline/Euler z żyrskopu - całkowanie/Calculate DCM_0 ==
  phi theta psi : Inport
  Rotation Angles to Direction Cosine Matrix : aerolibtransform2/Rotation Angles to Direction Cosine Matrix  rotationOrder=ZYX
  Selector : Selector  InputPortWidth=3  IndexOptions=Index vector (dialog)  Indices=[3 2 1]  OutputSizes=1
  DCM : Outport
  wires:
  Selector/1 -> Rotation Angles to Direction Cosine Matrix/1
  phi theta psi/1 -> Selector/1
  Rotation Angles to Direction Cosine Matrix/1 -> DCM/1

== system obliczeniaOffline/Euler z żyrskopu - całkowanie/Calculate Euer2 ==
  DCM : Inport
  Direction Cosine Matrix to Rotation Angles : aerolibtransform2/Direction Cosine Matrix to Rotation Angles  rotationOrder=ZYX  lim=Default
      settings: AttributesFormatString=Rotation Order: %<rotationOrder>
  Selector1 : Selector  InputPortWidth=3  IndexOptions=Index vector (dialog)  Indices=[3 2 1]  OutputSizes=1
  phi theta psi : Outport
  wires:
  Selector1/1 -> phi theta psi/1
  Direction Cosine Matrix to Rotation Angles/1 -> Selector1/1
  DCM/1 -> Direction Cosine Matrix to Rotation Angles/1

== system obliczeniaOffline/Euler z żyrskopu - całkowanie/Calculate Euler ==
  p q r : Inport
  reset : Inport  Port=2
  initialAngles : Inport  Port=3
  Discrete-Time Integrator1 : DiscreteIntegrator  ExternalReset=either  InitialConditionSource=external  InitialCondition=eul_0  SampleTime=-1  ICPrevOutput=DiscIntNeverNeededParam  ICPrevScaledInput=DiscIntNeverNeededParam
  phidot thetadot psidot : Subsystem
  Euler : Outport
  wires:
  p q r/1 -> phidot thetadot psidot/1(p q r)
  phidot thetadot psidot/1(phidot thetadot psi) -> Discrete-Time Integrator1/1
  Discrete-Time Integrator1/1 -> phidot thetadot psidot/2(phi theta psi), Euler/1
  reset/1 -> Discrete-Time Integrator1/2
  initialAngles/1 -> Discrete-Time Integrator1/3

== system obliczeniaOffline/Integrate with high-pass filters/Highpass Filter2 ==
  In : Inport
  Generated Filter Block : dsparch4/Biquad Filter  Tag=BlockMethodSubSystem  IIRFiltStruct=Direct form II  CoeffSource=Specify via dialog  BiQuadCoeffs=[1.9999999999999998 -1.9999891140812491 0 1 -0.98746704639308547 0]  a0Flag=Warning  IC=0  ICnum=0  ICden=0  InputProcessing=Columns as channels (frame based)  denAccumFracLength=30  denProdOutputFracLength=30  secondMemoryFracLength=15  roundingMode=Floor  overflowMode=off  ScaleValues=[0.012532953606914534;51.489014392199728]  optimizeScaleValues=off  ScaleValueMode=Specify via input port (g)  scaleValueFracLength=14  FilterSource=Specify via dialog  dfiltObjectName=dfilt.df2tsos([1 0.3 0.4],[1 0.1 0.2])
  Out : Outport
  wires:
  Generated Filter Block/1 -> Out/1
  In/1 -> Generated Filter Block/1

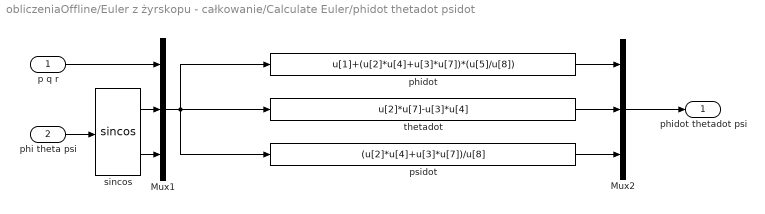
== system obliczeniaOffline/Euler z żyrskopu - całkowanie/Calculate Euler/phidot thetadot psidot ==
  p q r : Inport
  phi theta psi : Inport  Port=2
  Mux1 : Mux  Inputs=[3 3 3]
  Mux2 : Mux  Inputs=3
  phidot : Fcn  Expr=u[1]+(u[2]*u[4]+u[3]*u[7])*(u[5]/u[8])
  psidot : Fcn  Expr=(u[2]*u[4]+u[3]*u[7])/u[8]
  sincos : Trigonometry  Operator=sincos
  thetadot : Fcn  Expr=u[2]*u[7]-u[3]*u[4]
  phidot thetadot psi : Outport  InitialOutput=0
  wires:
  phi theta psi/1 -> sincos/1
  psidot/1 -> Mux2/3
  thetadot/1 -> Mux2/2
  sincos/1 -> Mux1/2
  p q r/1 -> Mux1/1
  sincos/2 -> Mux1/3
  Mux2/1 -> phidot thetadot psi/1
  phidot/1 -> Mux2/1
  Mux1/1 -> phidot/1, psidot/1, thetadot/1
